simulink model "Ejemplo01"  (R2021b)
settings: Solver=VariableStepAuto  StartTime=1  StopTime=10  RelTol=1e-3
settings Model: Creator=juandiegocastropadilla  LastModifiedBy=juandiegocastropadilla

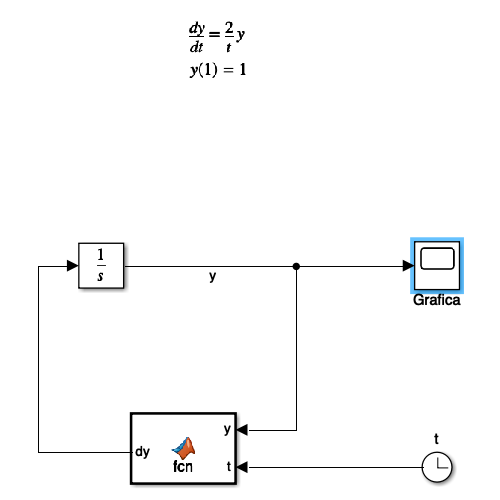
[thumbnail: Simulink's stored preview of the top-level diagram]
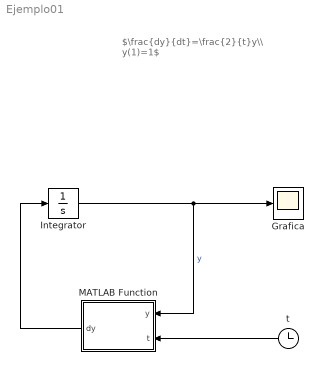
== system Ejemplo01 ==
  note: $\frac{dy}{dt}=\frac{2}{t}y\\ y(1)=1$
  Grafica : Scope
  Integrator : Integrator  InitialCondition=1
  MATLAB Function : MATLAB Function  TreatAsAtomicUnit=on
  t : Clock
  wires:
  Integrator/1 -> Grafica/1, MATLAB Function/1(y)  "y"
  MATLAB Function/1(dy) -> Integrator/1
  t/1 -> MATLAB Function/2(t)

== matlab function Ejemplo01/MATLAB Function ==
  data: y input; dy output; t input
function dy = fcn(y, t)

dy = ((2)/(t))*y;
